simulink model "PVarray_OC"  (R2021a)
settings: Solver=VariableStepAuto  StartTime=0.0  StopTime=80  MaxStep=0.1  RelTol=1e-3
libraries: spsDiodeLib x10, spsPVArrayLib x8, spsControlledVoltageSourceLib x1, spsCurrentMeasurementLib x1, simulink x1, spsVoltageMeasurementLib x1, spspowerguiLib x1
settings Model: Creator=Lenovo  LastModifiedBy=Lenovo

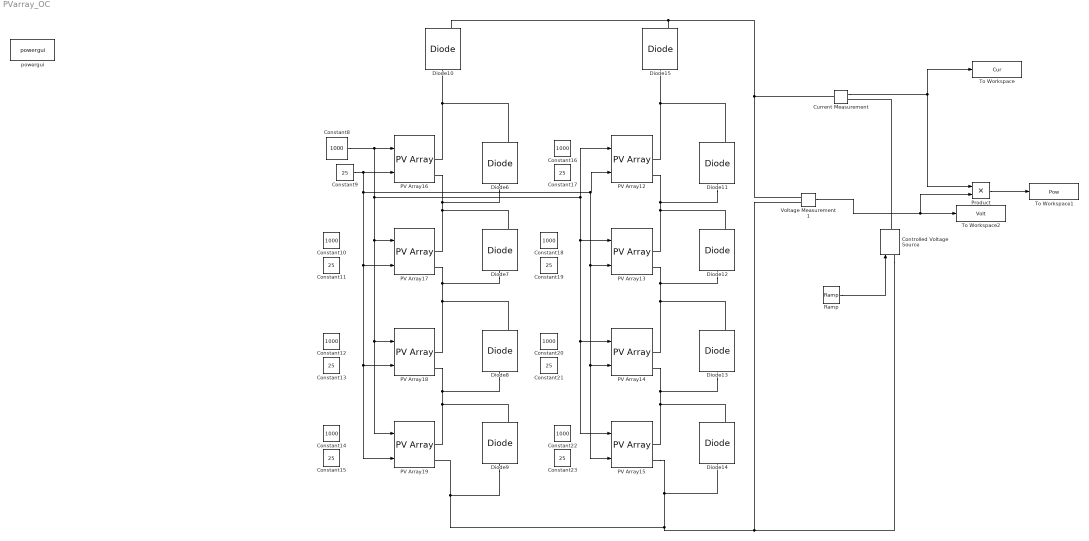
== system PVarray_OC ==
  Constant{8,10,12,14,16,18,20,22} (8 alike) : Constant  Value=1000
  Constant{9,11,13,15,17,19,21,23} (8 alike) : Constant  Value=25
  Controlled Voltage Source : spsControlledVoltageSourceLib/Controlled Voltage Source  Initialize=on  Source_Type=AC  Amplitude=0  Phase=0  Frequency=0  Measurements=None
  Current Measurement : spsCurrentMeasurementLib/Current Measurement  PhasorSimulation=off  OutputType=Complex  PSBequivalent=0
  Diode{6..15} (10 alike) : spsDiodeLib/Diode  Ron=0.001  Lon=0  Vf=0.8  IC=0  UseSnubber=0  Rs=500  Cs=250e-9  Measurements=on
  PV Array{12..19} (8 alike) : spsPVArrayLib/PV Array  Npar=1  Nser=1  PlotType=array @ 1000 W/m2 & specified temperatures  S_vec="[ 1000  500  100 ]"  Temp_C_vec="[ 45 25  ]"  ModuleName=User-defined  PlotWhenSelected=off  Pm=79.92  Ncell=36  Voc=21.6  Isc=4.89  Vm=18  Im=4.44  beta_Voc_pc=-0.34  alpha_Isc_pc=0.045  beta_Voc=-0.07344  alpha_Isc=0.0022005  IL=4.9034  I0=7.7859e-11  nI=0.94142  Rsh=76.2104  Rs=0.20928  RobustModel=off  RobustCellTemperature=313.3991  BAL=on  Tc=1e-6  Tfilter=5e-5
  Product : Product
  Ramp : simulink/Sources/Ramp  slope=1  start=0  InitialOutput=0
  To Workspace : ToWorkspace  VariableName=Cur  SaveFormat=Timeseries  SampleTime=-1
  To Workspace1 : ToWorkspace  VariableName=Pow  SaveFormat=Timeseries  SampleTime=-1
  To Workspace2 : ToWorkspace  VariableName=Volt  SaveFormat=Timeseries  SampleTime=-1
  Voltage Measurement1 : spsVoltageMeasurementLib/Voltage Measurement  PhasorSimulation=off  OutputType=Complex  PSBequivalent=0
  powergui : spspowerguiLib/powergui  Priority=1  SimulationMode=Continuous  SampleTime=50e-6  frequency=60  Iterations=50  frequencyindice=0  Pbase=100e6  ErrMax=1e-4  UnitsV=kV  UnitsW=MW  buscounter=0  FunctionMessages=off  echomessages=off  EnableUseOfTLC=off  CurrentSourceSwitches=off  DisableSnubberDevices=off  DisableRonSwitches=off  DisableVfSwitches=off  DisplayEquations=off  AutomaticDiscreteSolvers=off  SolverType=Tustin/Backward Euler (TBE)  Interpol=off  ExternalGateDelay=off  methode=off  Ts=100  x0status=blocks  SPID=on  SwTol=0  HookPort=off  NonlinearTolerance=1e-4  nMaxIteration=100  ContinueOnMaxIteration=off  RestoreLinks=warning  ResistiveCurrentMeasurement=off  Frange=[0:2:500]  Ylog=off  Xlog=on  ShowGrid=off  save=off  variable=ZData  structure=0  ZoomFFT=off  StartTime=0.0  cycles=1  DisplayStyle=1  fundamental=60  FreqAxis=off  MaxFrequency=1000  frequencyindicesteady=1  RmsSteady=1  display=off
  wires:
  Product/1 -> To Workspace1/1
  Voltage Measurement1/1 -> Product/2, To Workspace2/1
  Ramp/1 -> Controlled Voltage Source/1
  Current Measurement/1 -> Product/1, To Workspace/1
  Constant9/1 -> PV Array19/2, PV Array18/2, PV Array17/2, PV Array15/2, PV Array14/2, PV Array13/2, PV Array12/2, PV Array16/2
  Constant8/1 -> PV Array19/1, PV Array18/1, PV Array17/1, PV Array15/1, PV Array14/1, PV Array13/1, PV Array12/1, PV Array16/1
  connections:
  Diode9/LConn1 -- PV Array19/RConn2 -- Diode14/LConn1 -- PV Array15/RConn2 -- Controlled Voltage Source/LConn1 -- Voltage Measurement1/LConn2
  Diode10/LConn1 -- Diode6/RConn1 -- PV Array16/RConn1
  Diode15/RConn1 -- Current Measurement/LConn1 -- Voltage Measurement1/LConn1 -- Diode10/RConn1
  Diode12/LConn1 -- PV Array14/RConn1 -- Diode13/RConn1 -- PV Array13/RConn2
  Diode11/LConn1 -- PV Array12/RConn2 -- Diode12/RConn1 -- PV Array13/RConn1
  Diode13/LConn1 -- PV Array15/RConn1 -- Diode14/RConn1 -- PV Array14/RConn2
  Diode6/LConn1 -- PV Array16/RConn2 -- Diode7/RConn1 -- PV Array17/RConn1
  Diode7/LConn1 -- PV Array18/RConn1 -- Diode8/RConn1 -- PV Array17/RConn2
  Diode9/RConn1 -- PV Array18/RConn2 -- Diode8/LConn1 -- PV Array19/RConn1
  Diode15/LConn1 -- Diode11/RConn1 -- PV Array12/RConn1
  Controlled Voltage Source/RConn1 -- Current Measurement/RConn1
